simulink model "sxema"  (R2013a)
settings: Solver=ode45  StartTime=0.0  StopTime=20  RelTol=1e-3
undefined symbols (not defined in the file): K, T1, T2
settings Model: Creator=Huy Hung  LastModifiedBy=Huy Hung

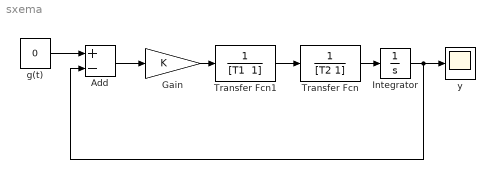
== system sxema ==
  Add : Sum  Inputs=+-
  Gain : Gain  Gain=K
  Integrator : Integrator  InitialCondition=1
  Transfer Fcn : TransferFcn  Denominator=[T2 1]
  Transfer Fcn1 : TransferFcn  Denominator="[T1  1]"
  g(t) : Constant  Value=0
  y : Scope
      settings: TimeRange=20  YMin=0  YMax=1.4  SampleInput=on
  wires:
  Transfer Fcn/1 -> Integrator/1
  Gain/1 -> Transfer Fcn1/1
  Transfer Fcn1/1 -> Transfer Fcn/1
  Integrator/1 -> y/1, Add/2
  g(t)/1 -> Add/1
  Add/1 -> Gain/1
